simulink model "Data_acquisition"  (R2024a)
settings: Solver=FixedStepDiscrete  StartTime=0.0  StopTime=inf  FixedStep=0.001  RelTol=1e-3  EnableMultiTasking=on
libraries: arduinosensorlib x2, arduinolib x2
settings Model: SimulationMode=external  ExtModeTrigDuration=2  Creator=mashr  LastModifiedBy=mashr
settings SolverCC: AutoInsertRateTranBlk=on
settings DataIOCC: DSMLogging=off  ReturnWorkspaceOutputs=off
settings OptimizationCC: EnhancedBackFolding=on  PassReuseOutputArgsAs=Individual arguments  ZeroExternalMemoryAtStartup=off  ZeroInternalMemoryAtStartup=off  MaxStackSize=64  OptimizeBlockOrder=speed  DifferentSizesBufferReuse=on  OptimizationCustomize=off  EfficientTunableParamExpr=on
settings DebuggingCC: ParameterTunabilityLossMsg=error
settings HardwareCC: ProdBitPerPointer=32  ProdBitPerSizeT=32  ProdBitPerPtrDiffT=32  ProdLargestAtomicInteger=Long  ProdLargestAtomicFloat=Double  ProdWordSize=32  ProdHWDeviceType=ARM Compatible->ARM Cortex
settings SFSimCC: MATLABDynamicMemAlloc=off
settings RTWCC: Description=Embedded Coder  SystemTargetFile=ert.tlc  HardwareBoard=ESP32-WROOM(Arduino Compatible)  TemplateMakefile=ert_default_tmf  Toolchain=ESP32  BuildConfiguration=Faster Runs
settings CodeAppCC: ForceParamTrailComments=on  IgnoreCustomStorageClasses=off  OperatorAnnotations=on  SimulinkDataObjDesc=on  SFDataObjDesc=on  InsertBlockDesc=on
settings ERTTargetCC: SupportContinuousTime=on  SupportVariableSizeSignals=on  ExtMode=on  ExtModeTransport=3  ExtModeStaticAlloc=on  ExtModeAutomaticAllocSize=off  ExtModeStaticAllocSize=65536  ExtModeMexFile=ext_xcp  ExtModeMexArgs=0 5 921600  ExtModeIntrfLevel=Level2 - Open

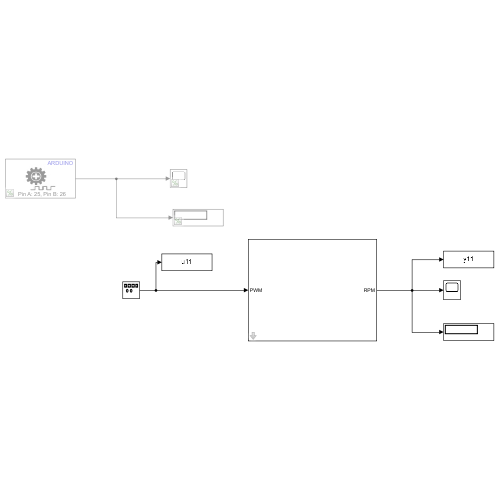
[thumbnail: Simulink's stored preview of the top-level diagram]
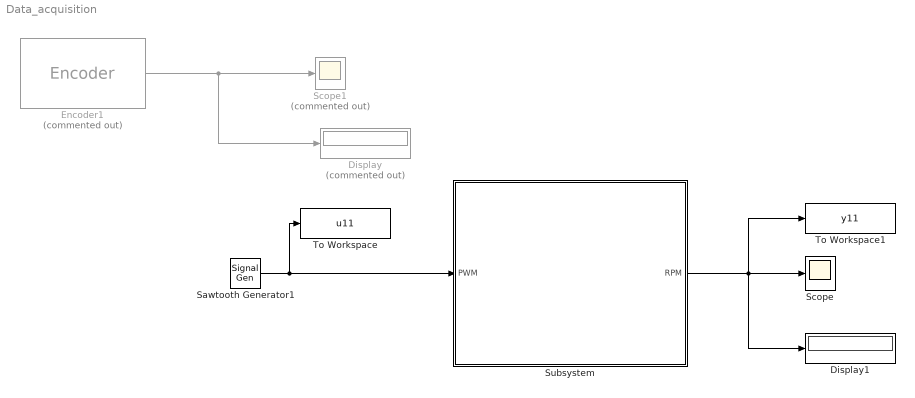
== system Data_acquisition ==
  Display : Display  Commented=on
  Display1 : Display
  Encoder1 : arduinosensorlib/Encoder  Commented=on  InputA=25  InputB=26  Mode=No reset  SampleTime=0.001
  Sawtooth Generator1 : SignalGenerator  WaveForm=sawtooth  Amplitude=255  Frequency=0.2
  Scope : Scope
  Scope1 : Scope  Commented=on
  Subsystem : Subsystem  mask{Ts=0.001}
      mask prompts: Ts "Sample Time"
  To Workspace : ToWorkspace  VariableName=u11  SaveFormat=Timeseries  SampleTime=0.001
      settings: Save2DSignal=2-D array (concatenate along first dimension)
  To Workspace1 : ToWorkspace  VariableName=y11  SaveFormat=Timeseries  SampleTime=0.001
      settings: Save2DSignal=2-D array (concatenate along first dimension)
  wires:
  Subsystem/1(RPM) -> Display1/1, Scope/1, To Workspace1/1
  Encoder1/1 -> Display/1, Scope1/1
  Sawtooth Generator1/1 -> To Workspace/1, Subsystem/1(PWM)

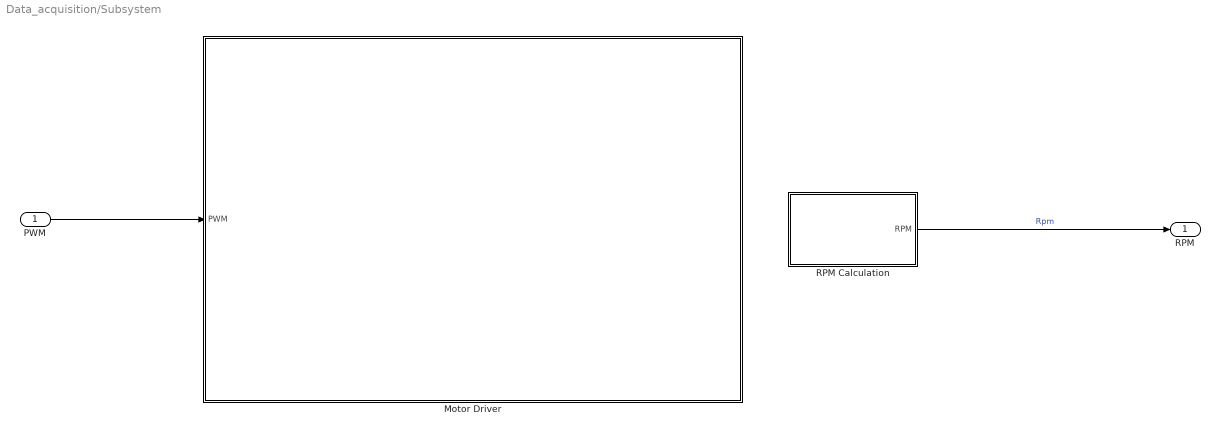
== system Data_acquisition/Subsystem ==
  PWM : Inport
  Motor Driver : Subsystem
  RPM Calculation : Subsystem
  RPM : Outport
  wires:
  PWM/1 -> Motor Driver/1(PWM)
  RPM Calculation/1(RPM) -> RPM/1  "Rpm"

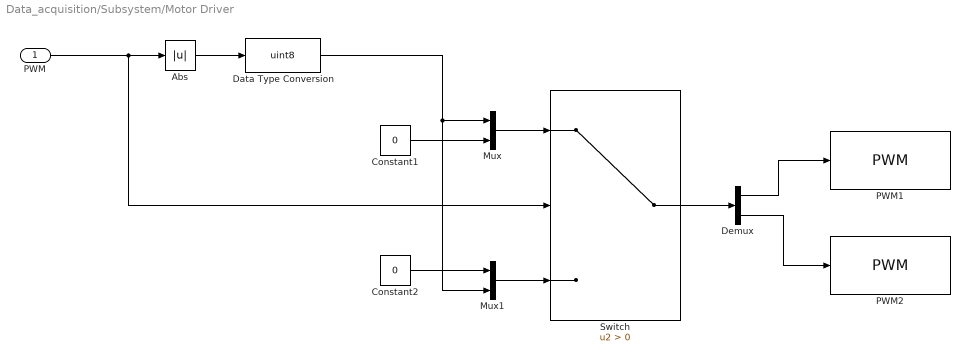
== system Data_acquisition/Subsystem/Motor Driver ==
  PWM : Inport
  Abs : Abs  SaturateOnIntegerOverflow=off
  Constant1 : Constant  Value=0  OutDataTypeStr=uint8
  Constant2 : Constant  Value=0  OutDataTypeStr=uint8
  Data Type Conversion : DataTypeConversion  OutDataTypeStr=uint8  SaturateOnIntegerOverflow=off  RndMeth=Floor
  Demux : Demux  Outputs=2
  Mux : Mux  Inputs=2
  Mux1 : Mux  Inputs=2
  PWM1 : arduinolib/PWM  pinNumber=33  frequencyType=Specify  desiredFrequency=16000  achievableFrequency=16000
  PWM2 : arduinolib/PWM  pinNumber=32  frequencyType=Specify  desiredFrequency=16000  achievableFrequency=16000
  Switch : Switch  Criteria=u2 > Threshold  SaturateOnIntegerOverflow=off  InputSameDT=off
  wires:
  Mux/1 -> Switch/1
  Switch/1 -> Demux/1
  Constant2/1 -> Mux1/1
  Constant1/1 -> Mux/2
  Mux1/1 -> Switch/3
  Demux/2 -> PWM2/1
  PWM/1 -> Switch/2, Abs/1
  Demux/1 -> PWM1/1
  Abs/1 -> Data Type Conversion/1
  Data Type Conversion/1 -> Mux1/2, Mux/1

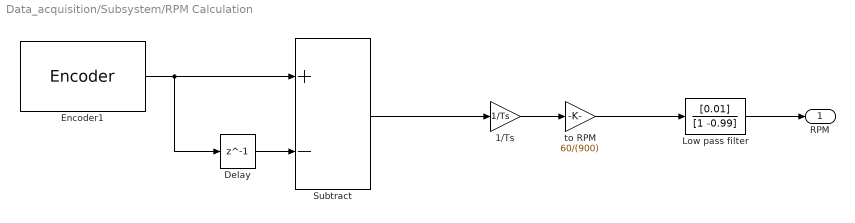
== system Data_acquisition/Subsystem/RPM Calculation ==
  1/Ts : Gain  Gain=1/Ts
  Delay : Delay  DelayLength=1  SampleTime=Ts
  Encoder1 : arduinosensorlib/Encoder  InputA=25  InputB=26  Mode=No reset  SampleTime=Ts
  Low pass filter : DiscreteFilter  Numerator=[0.01]  Denominator=[1 -0.99]
  Subtract : Sum  Inputs=+-
  to RPM : Gain  Gain=60/(900)  OutDataTypeStr=double
  RPM : Outport
  wires:
  Encoder1/1 -> Delay/1, Subtract/1
  Delay/1 -> Subtract/2
  Subtract/1 -> 1/Ts/1
  1/Ts/1 -> to RPM/1
  Low pass filter/1 -> RPM/1
  to RPM/1 -> Low pass filter/1
